simulink model "orion_casestudy_8"  (R2023a)
settings: Solver=VariableStepAuto  StartTime=0.0  StopTime=30  RelTol=1e-3
InitFcn:
  | RandStream.setGlobalStream(RandStream('mt19937ar','seed',sum(100*clock)));
undefined symbols (not defined in the file or in its folder): m, n
(part 3 of 3)

== stateflow chart orion_casestudy_8/DelaySwitch26 ==
  state Operation
  state Sending
  (default) -> Operation : {i=0;}
  (junction 7) -> Operation [order 2]
  Sending -> Operation : after(delay_array(i),msec)
      | {receive(inMsg);outMsg.data=0;send(outMsg);}
  Operation -> (junction 7) : inMsg{i = i + 1;}
  (junction 7) -> Sending [order 1] : [switch_array(i)==0]
  data: switch_array input; delay_array input; outMsg output; inMsg input; i local

== stateflow chart orion_casestudy_8/DelaySwitch27 ==
  state Operation
  state Sending
  (default) -> Operation : {i=0;}
  (junction 7) -> Operation [order 2]
  Sending -> Operation : after(delay_array(i),msec)
      | {receive(inMsg);outMsg.data=0;send(outMsg);}
  Operation -> (junction 7) : inMsg{i = i + 1;}
  (junction 7) -> Sending [order 1] : [switch_array(i)==0]
  data: switch_array input; delay_array input; outMsg output; inMsg input; i local

== stateflow chart orion_casestudy_8/DelaySwitch28 ==
  state Operation
  state Sending
  (default) -> Operation : {i=0;}
  (junction 7) -> Operation [order 2]
  Sending -> Operation : after(delay_array(i),msec)
      | {receive(inMsg);outMsg.data=0;send(outMsg);}
  Operation -> (junction 7) : inMsg{i = i + 1;}
  (junction 7) -> Sending [order 1] : [switch_array(i)==0]
  data: switch_array input; delay_array input; outMsg output; inMsg input; i local

== stateflow chart orion_casestudy_8/DelaySwitch29 ==
  state Operation
  state Sending
  (default) -> Operation : {i=0;}
  (junction 7) -> Operation [order 2]
  Sending -> Operation : after(delay_array(i),msec)
      | {receive(inMsg);outMsg.data=0;send(outMsg);}
  Operation -> (junction 7) : inMsg{i = i + 1;}
  (junction 7) -> Sending [order 1] : [switch_array(i)==0]
  data: switch_array input; delay_array input; outMsg output; inMsg input; i local

== stateflow chart orion_casestudy_8/DelaySwitch30 ==
  state Operation
  state Sending
  (default) -> Operation : {i=0;}
  (junction 7) -> Operation [order 2]
  Sending -> Operation : after(delay_array(i),msec)
      | {receive(inMsg);outMsg.data=0;send(outMsg);}
  Operation -> (junction 7) : inMsg{i = i + 1;}
  (junction 7) -> Sending [order 1] : [switch_array(i)==0]
  data: switch_array input; delay_array input; outMsg output; inMsg input; i local

== stateflow chart orion_casestudy_8/Master2 ==
  settings: updateMethod=CONTINUOUS
  state Connected
    entry:
    connStatus=2;
    state KeepAliveSendTimeout [parallel]
      settings: executionOrder=1
      state KeepAliveSend
      (default) -> KeepAliveSend
      KeepAliveSend -> KeepAliveSend [order 1] : after(delay_array(i)*5,msec)
          | {OrionKeepAliveOut.data=0;
          | send(OrionKeepAliveOut);
          | i = i + 1;}
      KeepAliveSend -> KeepAliveSend [order 2] : SendDataIn
          | {OrionAppDataOut.data=0;
          | send(OrionAppDataOut);}
    state KeepAliveRecieveTimeout [parallel]
      settings: executionOrder=2
      state KeepAlineRec
      (default) -> KeepAlineRec
      KeepAlineRec -> KeepAlineRec [order 2] : OrionKeepAliveIn
      KeepAlineRec -> KeepAlineRec [order 3] : OrionAppDataIn
  state Closed
    entry:
    connStatus=0;
  state Connecting
    entry:
    connStatus=1;
  Connected -> (junction 6) [order 1] : OrionConnConfIn
  (default) -> Closed : {i=1;}
  Connected -> (junction 6) [order 2] : OrionConnRespIn
  Connected -> (junction 6) [order 3] : OrionConnReqIn
  (junction 6) -> Closed
  KeepAlineRec -> Closed [order 1] : after(delay_array(i)*5,msec)
      | {i = i + 1;}
  Connecting -> (junction 36) [order 5] : OrionConnReqIn
  (junction 36) -> Closed
  Connecting -> (junction 36) [order 4] : OrionConnRespIn
  Connecting -> (junction 36) [order 2] : OrionKeepAliveIn
  Connecting -> Closed [order 3] : after(delay_array(i)*5,msec)
      | {i = i + 1;}
  Closed -> Connecting [order 2] : after(delay_array(i)*5,msec)
      | {OrionConnReqOut.data=0;send(OrionConnReqOut);i = i + 1;}
  Closed -> Connecting [order 1] : OrionConnReqIn
      | {OrionConnRespOut.data=0;send(OrionConnRespOut);}
  Connecting -> Connected [order 1] : OrionConnRespIn
      | {OrionConnConfOut.data=0;
      | send(OrionConnConfOut);}
  data: delay_array input; OrionKeepAliveOut output; OrionKeepAliveIn input; OrionConnConfOut output; OrionConnConfIn input; OrionConnRespOut output; OrionAppDataOut output; OrionAppDataIn input; OrionConnRespIn input; OrionConnReqIn input; OrionConnReqOut output; connStatus output; SendDataIn local; i local

== stateflow chart orion_casestudy_8/Slave2 ==
  settings: updateMethod=CONTINUOUS
  state Connected
    entry:
    connStatus=2;
    state KeepAliveSendTimeout [parallel]
      settings: executionOrder=1
      state KeepAliveSend
      (default) -> KeepAliveSend
      KeepAliveSend -> KeepAliveSend [order 1] : after(delay_array(i)*5,msec)
          |  {OrionKeepAliveOut.data=0;
          | send(OrionKeepAliveOut);i = i + 1;}
      KeepAliveSend -> KeepAliveSend [order 2] : SendDataIn
          | {OrionAppDataOut.data=0;
          | send(OrionAppDataOut);}
    state KeepAliveRecieveTimeout [parallel]
      settings: executionOrder=2
      state KeepAlineRec
      (default) -> KeepAlineRec
      KeepAlineRec -> KeepAlineRec [order 2] : OrionKeepAliveIn
      KeepAlineRec -> KeepAlineRec [order 3] : OrionAppDataIn
  state Closed
    entry:
    connStatus=0;
  state Connecting
    entry:
    connStatus=1;
  Connected -> (junction 6) [order 2] : OrionConnRespIn
  Connected -> (junction 6) [order 3] : OrionConnReqIn
  (default) -> Closed : {i=1;}
  (junction 6) -> Closed
  Connected -> (junction 6) [order 1] : OrionConnConfIn
  KeepAlineRec -> Closed [order 1] : after(delay_array(i)*5,msec)
      | {i = i + 1;}
  Connecting -> (junction 36) [order 6] : OrionAppDataIn
  Connecting -> (junction 36) [order 5] : OrionConnReqIn
  (junction 36) -> Closed
  Connecting -> (junction 36) [order 4] : OrionConnRespIn
  Connecting -> (junction 36) [order 3] : OrionKeepAliveIn
  Closed -> Connecting : OrionConnReqIn
      | {OrionConnRespOut.data=0;
      | send(OrionConnRespOut);}
  Connecting -> Closed [order 1] : after(delay_array(i)*5,msec)
      | {i = i + 1;}
  Connecting -> Connected [order 2] : OrionConnConfIn{OrionConnConfOut.data=0;send(OrionConnConfOut);}
  data: OrionKeepAliveIn input; OrionConnConfOut output; OrionConnRespOut output; OrionKeepAliveOut output; OrionAppDataOut output; OrionAppDataIn input; OrionConnRespIn input; OrionConnReqIn input; OrionConnReqOut output size=1; connStatus output; SendDataIn local; OrionConnConfIn input; delay_array input; i local

== stateflow chart orion_casestudy_8/DelaySwitch2 ==
  state Operation
  state Sending
  (default) -> Operation : {i=0;}
  (junction 7) -> Operation [order 2]
  Sending -> Operation : after(delay_array(i),msec)
      | {receive(inMsg);outMsg.data=0;send(outMsg);}
  Operation -> (junction 7) : inMsg{i = i + 1;}
  (junction 7) -> Sending [order 1] : [switch_array(i)==0]
  data: switch_array input; delay_array input; outMsg output; inMsg input; i local

== stateflow chart orion_casestudy_8/DelaySwitch31 ==
  state Operation
  state Sending
  (default) -> Operation : {i=0;}
  (junction 7) -> Operation [order 2]
  Sending -> Operation : after(delay_array(i),msec)
      | {receive(inMsg);outMsg.data=0;send(outMsg);}
  Operation -> (junction 7) : inMsg{i = i + 1;}
  (junction 7) -> Sending [order 1] : [switch_array(i)==0]
  data: switch_array input; delay_array input; outMsg output; inMsg input; i local

== stateflow chart orion_casestudy_8/DelaySwitch32 ==
  state Operation
  state Sending
  (default) -> Operation : {i=0;}
  (junction 7) -> Operation [order 2]
  Sending -> Operation : after(delay_array(i),msec)
      | {receive(inMsg);outMsg.data=0;send(outMsg);}
  Operation -> (junction 7) : inMsg{i = i + 1;}
  (junction 7) -> Sending [order 1] : [switch_array(i)==0]
  data: switch_array input; delay_array input; outMsg output; inMsg input; i local

== stateflow chart orion_casestudy_8/DelaySwitch33 ==
  state Operation
  state Sending
  (default) -> Operation : {i=0;}
  (junction 7) -> Operation [order 2]
  Sending -> Operation : after(delay_array(i),msec)
      | {receive(inMsg);outMsg.data=0;send(outMsg);}
  Operation -> (junction 7) : inMsg{i = i + 1;}
  (junction 7) -> Sending [order 1] : [switch_array(i)==0]
  data: switch_array input; delay_array input; outMsg output; inMsg input; i local

== stateflow chart orion_casestudy_8/DelaySwitch34 ==
  state Operation
  state Sending
  (default) -> Operation : {i=0;}
  (junction 7) -> Operation [order 2]
  Sending -> Operation : after(delay_array(i),msec)
      | {receive(inMsg);outMsg.data=0;send(outMsg);}
  Operation -> (junction 7) : inMsg{i = i + 1;}
  (junction 7) -> Sending [order 1] : [switch_array(i)==0]
  data: switch_array input; delay_array input; outMsg output; inMsg input; i local

== stateflow chart orion_casestudy_8/DelaySwitch35 ==
  state Operation
  state Sending
  (default) -> Operation : {i=0;}
  (junction 7) -> Operation [order 2]
  Sending -> Operation : after(delay_array(i),msec)
      | {receive(inMsg);outMsg.data=0;send(outMsg);}
  Operation -> (junction 7) : inMsg{i = i + 1;}
  (junction 7) -> Sending [order 1] : [switch_array(i)==0]
  data: switch_array input; delay_array input; outMsg output; inMsg input; i local

== stateflow chart orion_casestudy_8/DelaySwitch36 ==
  state Operation
  state Sending
  (default) -> Operation : {i=0;}
  (junction 7) -> Operation [order 2]
  Sending -> Operation : after(delay_array(i),msec)
      | {receive(inMsg);outMsg.data=0;send(outMsg);}
  Operation -> (junction 7) : inMsg{i = i + 1;}
  (junction 7) -> Sending [order 1] : [switch_array(i)==0]
  data: switch_array input; delay_array input; outMsg output; inMsg input; i local

== stateflow chart orion_casestudy_8/DelaySwitch37 ==
  state Operation
  state Sending
  (default) -> Operation : {i=0;}
  (junction 7) -> Operation [order 2]
  Sending -> Operation : after(delay_array(i),msec)
      | {receive(inMsg);outMsg.data=0;send(outMsg);}
  Operation -> (junction 7) : inMsg{i = i + 1;}
  (junction 7) -> Sending [order 1] : [switch_array(i)==0]
  data: switch_array input; delay_array input; outMsg output; inMsg input; i local

== stateflow chart orion_casestudy_8/DelaySwitch38 ==
  state Operation
  state Sending
  (default) -> Operation : {i=0;}
  (junction 7) -> Operation [order 2]
  Sending -> Operation : after(delay_array(i),msec)
      | {receive(inMsg);outMsg.data=0;send(outMsg);}
  Operation -> (junction 7) : inMsg{i = i + 1;}
  (junction 7) -> Sending [order 1] : [switch_array(i)==0]
  data: switch_array input; delay_array input; outMsg output; inMsg input; i local

== stateflow chart orion_casestudy_8/DelaySwitch39 ==
  state Operation
  state Sending
  (default) -> Operation : {i=0;}
  (junction 7) -> Operation [order 2]
  Sending -> Operation : after(delay_array(i),msec)
      | {receive(inMsg);outMsg.data=0;send(outMsg);}
  Operation -> (junction 7) : inMsg{i = i + 1;}
  (junction 7) -> Sending [order 1] : [switch_array(i)==0]
  data: switch_array input; delay_array input; outMsg output; inMsg input; i local

== stateflow chart orion_casestudy_8/Master ==
  settings: updateMethod=CONTINUOUS
  state Connected
    entry:
    connStatus=2;
    state KeepAliveSendTimeout [parallel]
      settings: executionOrder=1
      state KeepAliveSend
      (default) -> KeepAliveSend
      KeepAliveSend -> KeepAliveSend [order 1] : after(delay_array(i)*5,msec)
          | {OrionKeepAliveOut.data=0;
          | send(OrionKeepAliveOut);
          | i = i + 1;}
      KeepAliveSend -> KeepAliveSend [order 2] : SendDataIn
          | {OrionAppDataOut.data=0;
          | send(OrionAppDataOut);}
    state KeepAliveRecieveTimeout [parallel]
      settings: executionOrder=2
      state KeepAlineRec
      (default) -> KeepAlineRec
      KeepAlineRec -> KeepAlineRec [order 2] : OrionKeepAliveIn
      KeepAlineRec -> KeepAlineRec [order 3] : OrionAppDataIn
  state Closed
    entry:
    connStatus=0;
  state Connecting
    entry:
    connStatus=1;
  Connected -> (junction 6) [order 1] : OrionConnConfIn
  (default) -> Closed : {i=1;}
  Connected -> (junction 6) [order 2] : OrionConnRespIn
  Connected -> (junction 6) [order 3] : OrionConnReqIn
  (junction 6) -> Closed
  KeepAlineRec -> Closed [order 1] : after(delay_array(i)*5,msec)
      | {i = i + 1;}
  Connecting -> (junction 36) [order 5] : OrionConnReqIn
  (junction 36) -> Closed
  Connecting -> (junction 36) [order 4] : OrionConnRespIn
  Connecting -> (junction 36) [order 2] : OrionKeepAliveIn
  Connecting -> Closed [order 3] : after(delay_array(i)*5,msec)
      | {i = i + 1;}
  Closed -> Connecting [order 2] : after(delay_array(i)*5,msec)
      | {OrionConnReqOut.data=0;send(OrionConnReqOut);i = i + 1;}
  Closed -> Connecting [order 1] : OrionConnReqIn
      | {OrionConnRespOut.data=0;send(OrionConnRespOut);}
  Connecting -> Connected [order 1] : OrionConnRespIn
      | {OrionConnConfOut.data=0;
      | send(OrionConnConfOut);}
  data: delay_array input; OrionKeepAliveOut output; OrionKeepAliveIn input; OrionConnConfOut output; OrionConnConfIn input; OrionConnRespOut output; OrionAppDataOut output; OrionAppDataIn input; OrionConnRespIn input; OrionConnReqIn input; OrionConnReqOut output; connStatus output; SendDataIn local; i local

== stateflow chart orion_casestudy_8/DelaySwitch40 ==
  state Operation
  state Sending
  (default) -> Operation : {i=0;}
  (junction 7) -> Operation [order 2]
  Sending -> Operation : after(delay_array(i),msec)
      | {receive(inMsg);outMsg.data=0;send(outMsg);}
  Operation -> (junction 7) : inMsg{i = i + 1;}
  (junction 7) -> Sending [order 1] : [switch_array(i)==0]
  data: switch_array input; delay_array input; outMsg output; inMsg input; i local

== stateflow chart orion_casestudy_8/Master3 ==
  settings: updateMethod=CONTINUOUS
  state Connected
    entry:
    connStatus=2;
    state KeepAliveSendTimeout [parallel]
      settings: executionOrder=1
      state KeepAliveSend
      (default) -> KeepAliveSend
      KeepAliveSend -> KeepAliveSend [order 1] : after(delay_array(i)*5,msec)
          | {OrionKeepAliveOut.data=0;
          | send(OrionKeepAliveOut);
          | i = i + 1;}
      KeepAliveSend -> KeepAliveSend [order 2] : SendDataIn
          | {OrionAppDataOut.data=0;
          | send(OrionAppDataOut);}
    state KeepAliveRecieveTimeout [parallel]
      settings: executionOrder=2
      state KeepAlineRec
      (default) -> KeepAlineRec
      KeepAlineRec -> KeepAlineRec [order 2] : OrionKeepAliveIn
      KeepAlineRec -> KeepAlineRec [order 3] : OrionAppDataIn
  state Closed
    entry:
    connStatus=0;
  state Connecting
    entry:
    connStatus=1;
  Connected -> (junction 6) [order 1] : OrionConnConfIn
  (default) -> Closed : {i=1;}
  Connected -> (junction 6) [order 2] : OrionConnRespIn
  Connected -> (junction 6) [order 3] : OrionConnReqIn
  (junction 6) -> Closed
  KeepAlineRec -> Closed [order 1] : after(delay_array(i)*5,msec)
      | {i = i + 1;}
  Connecting -> (junction 36) [order 5] : OrionConnReqIn
  (junction 36) -> Closed
  Connecting -> (junction 36) [order 4] : OrionConnRespIn
  Connecting -> (junction 36) [order 2] : OrionKeepAliveIn
  Connecting -> Closed [order 3] : after(delay_array(i)*5,msec)
      | {i = i + 1;}
  Closed -> Connecting [order 2] : after(delay_array(i)*5,msec)
      | {OrionConnReqOut.data=0;send(OrionConnReqOut);i = i + 1;}
  Closed -> Connecting [order 1] : OrionConnReqIn
      | {OrionConnRespOut.data=0;send(OrionConnRespOut);}
  Connecting -> Connected [order 1] : OrionConnRespIn
      | {OrionConnConfOut.data=0;
      | send(OrionConnConfOut);}
  data: delay_array input; OrionKeepAliveOut output; OrionKeepAliveIn input; OrionConnConfOut output; OrionConnConfIn input; OrionConnRespOut output; OrionAppDataOut output; OrionAppDataIn input; OrionConnRespIn input; OrionConnReqIn input; OrionConnReqOut output; connStatus output; SendDataIn local; i local
